simulink model "FieldOrientedController"  (R2020a)
settings: configuration reference "SLRT" (kept outside this file)
undefined symbols (not defined in the file): paramAdcAmperePerTransducerVolt, paramAdcTransducerVoltAtZeroAmpere, paramCurrentControlI, paramCurrentControlP, paramCurrentControlSatVoltage, paramEncoderCalibrationDuration, paramEncoderCalibrationMaxError, paramEncoderCalibrationVoltage, paramEncoderRotorPositionAtZeroCount, paramEncoderRotorPositionPerCount, paramOpenLoopVelocityAcceleration, paramOpenLoopVelocityToVoltsBias, paramOpenLoopVelocityToVoltsScalar, paramOverCurrentDuration, paramOverCurrentEnable, paramOverCurrentLimit, paramPwmCompareAtZeroVolt, paramPwmCompareMax, paramPwmComparePerVolt, paramVelocityControlI, paramVelocityControlP, paramVelocityControlSatCurrent, paramVelocityFilterCoeffDen, paramVelocityFilterCoeffNum, PolePairs, sampleTime
libraries: simulink x5
(part 2 of 2)

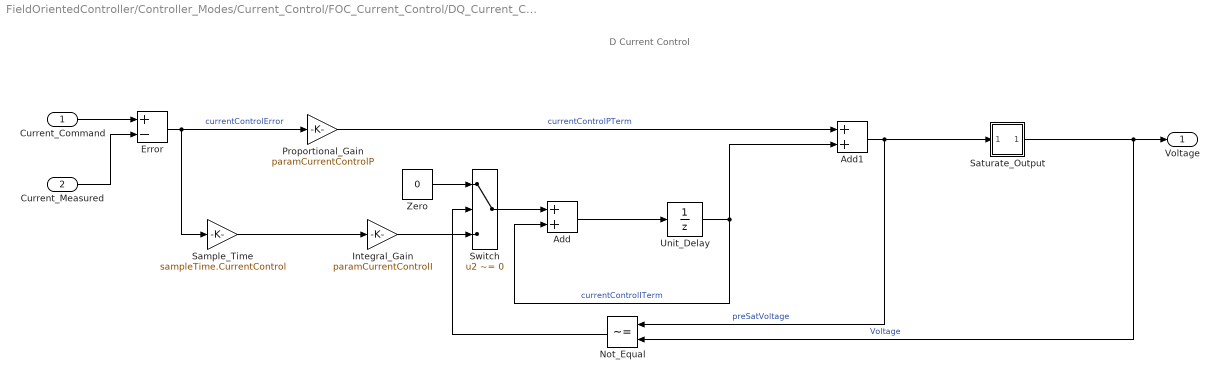
== system FieldOrientedController/Controller_Modes/Current_Control/FOC_Current_Control/DQ_Current_Control/D_Current_Control ==
  note: D Current Control
  Current_Command : Inport
  Current_Measured : Inport  Port=2
  Add : Sum
  Add1 : Sum
  Error : Sum  Inputs=+-
  Integral_Gain : Gain  Gain=paramCurrentControlI
      settings: AttributesFormatString=|
      | -----------------------------------
      | Gain = %<Gain>
  Not_Equal : RelationalOperator  Operator=~=  OutDataTypeStr=boolean  RndMeth=Nearest
  Proportional_Gain : Gain  Gain=paramCurrentControlP
      settings: AttributesFormatString=|
      | -----------------------------------
      | Gain = %<Gain>
  Sample_Time : Gain  Gain=sampleTime.CurrentControl
      settings: AttributesFormatString=|
      | -----------------------------------
      | Gain = %<Gain>
  Saturate_Output : Subsystem  mask(Saturate Magnitude){magnitudeLimit=paramCurrentControlSatVoltage}
      mask prompts: magnitudeLimit "Magnitude limit:"
      mask help:
      | Saturates input where:
      |    Upper limit =   Magnitude limit
      |    Lower limit = - Magnitude limit
      settings: AttributesFormatString=|
      | --------------------------------------------
      | Upper limit = %<magnitudeLimit>
      | Lower limit = -%<magnitudeLimit>
      mask Display: plot([0.15 0.85],[.5 .5],[.5 .5],[0.05 0.95],0.15+0.7*[0 .25 .75 1],0.05+0.9*[.25 .25 .75 .75]);
  Switch : Switch  Criteria=u2 ~= 0
  Unit_Delay : UnitDelay  SampleTime=-1  HasFrameUpgradeWarning=on
  Zero : Constant  Value=0  OutDataTypeStr=Inherit: Inherit via back propagation
  Voltage : Outport  VectorParamsAs1DForOutWhenUnconnected=off
  wires:
  Integral_Gain/1 -> Switch/3
  Unit_Delay/1 -> Add/2, Add1/2  "currentControlITerm"
  Sample_Time/1 -> Integral_Gain/1
  Add/1 -> Unit_Delay/1
  Not_Equal/1 -> Switch/2
  Proportional_Gain/1 -> Add1/1  "currentControlPTerm"
  Current_Measured/1 -> Error/2
  Switch/1 -> Add/1
  Saturate_Output/1(Out) -> Voltage/1, Not_Equal/2  "Voltage"
  Error/1 -> Proportional_Gain/1, Sample_Time/1  "currentControlError"
  Current_Command/1 -> Error/1
  Zero/1 -> Switch/1
  Add1/1 -> Not_Equal/1, Saturate_Output/1(In)  "preSatVoltage"

== system FieldOrientedController/Controller_Modes/Current_Control/FOC_Current_Control/DQ_Current_Control/Q_Current_Control ==
  note: Q Current Control
  Current_Command : Inport
  Current_Measured : Inport  Port=2
  Add : Sum
  Add1 : Sum
  Error : Sum  Inputs=+-
  Integral_Gain : Gain  Gain=paramCurrentControlI
      settings: AttributesFormatString=|
      | -----------------------------------
      | Gain = %<Gain>
  Not_Equal : RelationalOperator  Operator=~=  OutDataTypeStr=boolean  RndMeth=Nearest
  Proportional_Gain : Gain  Gain=paramCurrentControlP
      settings: AttributesFormatString=|
      | -----------------------------------
      | Gain = %<Gain>
  Sample_Time : Gain  Gain=sampleTime.CurrentControl
      settings: AttributesFormatString=|
      | -----------------------------------
      | Gain = %<Gain>
  Saturate_Output : Subsystem  mask(Saturate Magnitude){magnitudeLimit=paramCurrentControlSatVoltage}
      mask prompts: magnitudeLimit "Magnitude limit:"
      mask help:
      | Saturates input where:
      |    Upper limit =   Magnitude limit
      |    Lower limit = - Magnitude limit
      settings: AttributesFormatString=|
      | --------------------------------------------
      | Upper limit = %<magnitudeLimit>
      | Lower limit = -%<magnitudeLimit>
      mask Display: plot([0.15 0.85],[.5 .5],[.5 .5],[0.05 0.95],0.15+0.7*[0 .25 .75 1],0.05+0.9*[.25 .25 .75 .75]);
  Switch : Switch  Criteria=u2 ~= 0
  Unit_Delay : UnitDelay  SampleTime=-1  HasFrameUpgradeWarning=on
  Zero : Constant  Value=0  OutDataTypeStr=Inherit: Inherit via back propagation
  Voltage : Outport  VectorParamsAs1DForOutWhenUnconnected=off
  wires:
  Saturate_Output/1(Out) -> Voltage/1, Not_Equal/2  "Voltage"
  Add1/1 -> Not_Equal/1, Saturate_Output/1(In)  "preSatVoltage"
  Current_Measured/1 -> Error/2
  Unit_Delay/1 -> Add/2, Add1/2  "currentControlITerm"
  Proportional_Gain/1 -> Add1/1  "currentControlPTerm"
  Zero/1 -> Switch/1
  Error/1 -> Proportional_Gain/1, Sample_Time/1  "currentControlError"
  Sample_Time/1 -> Integral_Gain/1
  Current_Command/1 -> Error/1
  Add/1 -> Unit_Delay/1
  Integral_Gain/1 -> Switch/3
  Not_Equal/1 -> Switch/2
  Switch/1 -> Add/1

== system FieldOrientedController/Controller_Modes/Open_Loop_Velocity_Control/Open_Loop_Velocity_Control/Electrical_Velocity_To_Position/Mod_Two_Pi_Once ==
  note: Mod Two Pi Once
  X : Inport
  Add1 : Sum  Inputs=+-
  Add2 : Sum
  Greater_Than : RelationalOperator  OutDataTypeStr=boolean  RndMeth=Nearest
  Input_Range : SignalSpecification  OutMin=-4*pi  OutMax=4*pi
      settings: AttributesFormatString=|
      | -----------------------
      | Min = %<OutMin>
      | Max = %<OutMax>
  Less_Than : RelationalOperator  Operator=<  OutDataTypeStr=boolean  RndMeth=Nearest
  Output_Range : SignalSpecification  OutMin=0  OutMax=2*pi
      settings: AttributesFormatString=|
      | -----------------------
      | Min = %<OutMin>
      | Max = %<OutMax>
  Switch : Switch  Criteria=u2 ~= 0  InputSameDT=on
  Switch1 : Switch  Criteria=u2 ~= 0  InputSameDT=on
  Two_Pi : Constant  Value=2*pi  OutDataTypeStr=Inherit: Inherit via back propagation
  Two_Pi1 : Constant  Value=2*pi  OutDataTypeStr=Inherit: Inherit via back propagation
  Two_Pi2 : Constant  Value=2*pi  OutDataTypeStr=Inherit: Inherit via back propagation
  Zero : Constant  Value=0  OutDataTypeStr=Inherit: Inherit via back propagation
  Mod_X_Two_Pi : Outport  VectorParamsAs1DForOutWhenUnconnected=off
  wires:
  Output_Range/1 -> Mod_X_Two_Pi/1
  Zero/1 -> Less_Than/2
  Two_Pi2/1 -> Add2/2
  Add2/1 -> Switch1/1
  Less_Than/1 -> Switch1/2
  Switch1/1 -> Switch/3
  Two_Pi1/1 -> Greater_Than/2
  Two_Pi/1 -> Add1/2
  Add1/1 -> Switch/1
  Greater_Than/1 -> Switch/2
  X/1 -> Input_Range/1
  Switch/1 -> Output_Range/1
  Input_Range/1 -> Add1/1, Greater_Than/1, Add2/1, Less_Than/1, Switch1/3

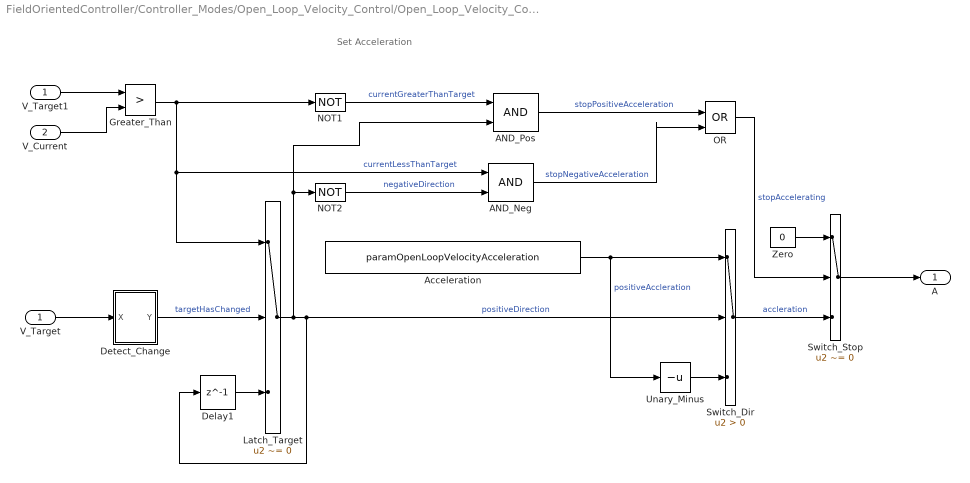
== system FieldOrientedController/Controller_Modes/Open_Loop_Velocity_Control/Open_Loop_Velocity_Control/Ramp_Velocity/Set_Acceleration ==
  note: Set Acceleration
  V_Target : Inport
  V_Current : Inport  Port=2
  AND_Neg : Logic  IconShape=distinctive  AllPortsSameDT=off  OutDataTypeStr=boolean
  AND_Pos : Logic  IconShape=distinctive  AllPortsSameDT=off  OutDataTypeStr=boolean
  Acceleration : Constant  Value=paramOpenLoopVelocityAcceleration  OutDataTypeStr=Inherit: Inherit via back propagation  SampleTime=-1
  Delay1 : Delay  DelayLength=1
  Detect_Change : Subsystem
  Greater_Than : RelationalOperator  Operator=>  OutDataTypeStr=boolean  RndMeth=Nearest
  Latch_Target : Switch  Criteria=u2 ~= 0
  NOT1 : Logic  Operator=NOT  IconShape=distinctive  AllPortsSameDT=off  OutDataTypeStr=boolean
  NOT2 : Logic  Operator=NOT  IconShape=distinctive  AllPortsSameDT=off  OutDataTypeStr=boolean
  OR : Logic  Operator=OR  IconShape=distinctive  AllPortsSameDT=off  OutDataTypeStr=boolean
  Switch_Dir : Switch  Criteria=u2 > Threshold
  Switch_Stop : Switch  Criteria=u2 ~= 0
  Unary_Minus : UnaryMinus
  V_Target1 : InportShadow
  Zero : Constant  Value=0  OutDataTypeStr=Inherit: Inherit via back propagation  SampleTime=-1
  A : Outport  VectorParamsAs1DForOutWhenUnconnected=off
  wires:
  AND_Neg/1 -> OR/2  "stopNegativeAcceleration"
  NOT2/1 -> AND_Neg/2  "negativeDirection"
  OR/1 -> Switch_Stop/2  "stopAccelerating"
  AND_Pos/1 -> OR/1  "stopPositiveAcceleration"
  NOT1/1 -> AND_Pos/1  "currentGreaterThanTarget"
  Zero/1 -> Switch_Stop/1
  Switch_Dir/1 -> Switch_Stop/3  "accleration"
  Switch_Stop/1 -> A/1
  Acceleration/1 -> Switch_Dir/1, Unary_Minus/1  "positiveAccleration"
  Unary_Minus/1 -> Switch_Dir/3
  Detect_Change/1(Y) -> Latch_Target/2  "targetHasChanged"
  V_Target/1 -> Detect_Change/1(X)
  V_Target1/1 -> Greater_Than/1
  V_Current/1 -> Greater_Than/2
  Delay1/1 -> Latch_Target/3
  Greater_Than/1 -> AND_Neg/1, Latch_Target/1, NOT1/1  "currentLessThanTarget"
  Latch_Target/1 -> Delay1/1, Switch_Dir/2, NOT2/1, AND_Pos/2  "positiveDirection"

== system FieldOrientedController/Controller_Modes/Current_Control/FOC_Current_Control/DQ_Current_Control/D_Current_Control/Saturate_Output ==
  note: Saturate Magnitude Library
  In : Inport
  Negate : UnaryMinus
  Saturation_Dynamic : simulink/Discontinuities/Saturation Dynamic  OutMin=[]  OutMax=[]  OutDataTypeStr=Inherit: Same as second input  OutDataType=fixdt(1, 16)  OutScaling=2^-10  DoSatur=off
  Saturation_Magntidue : Constant  Value=magnitudeLimit  OutDataTypeStr=Inherit: Inherit via back propagation
  Out : Outport  VectorParamsAs1DForOutWhenUnconnected=off
  wires:
  Saturation_Magntidue/1 -> Negate/1, Saturation_Dynamic/1
  Saturation_Dynamic/1 -> Out/1
  Negate/1 -> Saturation_Dynamic/3
  In/1 -> Saturation_Dynamic/2

== system FieldOrientedController/Controller_Modes/Current_Control/FOC_Current_Control/DQ_Current_Control/Q_Current_Control/Saturate_Output ==
  note: Saturate Magnitude Library
  In : Inport
  Negate : UnaryMinus
  Saturation_Dynamic : simulink/Discontinuities/Saturation Dynamic  OutMin=[]  OutMax=[]  OutDataTypeStr=Inherit: Same as second input  OutDataType=fixdt(1, 16)  OutScaling=2^-10  DoSatur=off
  Saturation_Magntidue : Constant  Value=magnitudeLimit  OutDataTypeStr=Inherit: Inherit via back propagation
  Out : Outport  VectorParamsAs1DForOutWhenUnconnected=off
  wires:
  Saturation_Magntidue/1 -> Negate/1, Saturation_Dynamic/1
  Saturation_Dynamic/1 -> Out/1
  Negate/1 -> Saturation_Dynamic/3
  In/1 -> Saturation_Dynamic/2

== system FieldOrientedController/Controller_Modes/Open_Loop_Velocity_Control/Open_Loop_Velocity_Control/Ramp_Velocity/Set_Acceleration/Detect_Change ==
  note: Detect Change
  X : Inport
  Add : Sum  Inputs=+-
  Delay : Delay  DelayLength=1
  Not_Equal_Zero : simulink/Logic and Bit Operations/Compare To Zero  relop=~=  OutDataTypeStr=boolean
  Y : Outport  VectorParamsAs1DForOutWhenUnconnected=off
  wires:
  Delay/1 -> Add/2
  Add/1 -> Not_Equal_Zero/1
  Not_Equal_Zero/1 -> Y/1
  X/1 -> Add/1, Delay/1

== stateflow chart FieldOrientedController/Controller_Modes/Over_Current_Detector/Detect_Over_Current_Error ==
  note: Detect Over Current Error
  note: If either Phase A Current (current[0]) or Phase B Current are above the threshold for a given duration, generate an error.
      | The error is reset when over current detection is disabled.
  state Error
    entry:
    error = true;
  state No_Error
    entry:
    error = false;
  state Wait_For_Reset
  (default) -> No_Error
  No_Error -> Error : [enableOverCurrentDetect && ...
      |  duration((phaseCurrentA >= paramOverCurrentLimit) || ...
      | (phaseCurrentB >= paramOverCurrentLimit))>paramOverCurrentDuration]
  Wait_For_Reset -> No_Error : [enableOverCurrentDetect]
  Error -> Wait_For_Reset : [~enableOverCurrentDetect]
  data: enableOverCurrentDetect input; phaseCurrentA input; phaseCurrentB input; error output boolean; paramOverCurrentDuration parameter; paramOverCurrentLimit parameter

== matlab function FieldOrientedController/EncoderToPositionAndVelocity/Position_Delta_To_Velocity/Rotor_Position_Delta_To_Velocity ==
  settings: fimath=|
      | fimath(...
      |     'RoundingMethod','Floor',...
      |     'OverflowAction','Wrap',...
      |     'ProductMode','KeepLSB',...
      |     'ProductWordLength',32,...
      |     'SumMode','KeepLSB',...
      |     'SumWordLength',32)
  data: positionDelta input; rotorVelocity output; positionDeltaBufferLength parameter; sampleFrequency parameter
function rotorVelocity = fcn(...                        %#codegen
                          positionDelta,...             % Input
                          positionDeltaBufferLength,... % Constant parameter
                          sampleFrequency)              % Constant parameter
% Copyright 2014 The MathWorks, Inc.

%% States
persistent positionDeltaBuffer;
persistent bufferIndex;

%% Constraints
assert(log2(positionDeltaBufferLength) == floor(log2(positionDeltaBufferLength)),...
    'Delay buffer must be a power of two.');

%% Initialize states
if isempty(positionDeltaBuffer)
    positionDeltaBuffer = ...
           zeros(positionDeltaBufferLength,1,...
                 'like', positionDelta);
    bufferIndex = int32(0);
end

%% Initialize constants
bufferIndexBitMask = positionDeltaBufferLength - 1;
reciprocalOfBufferLength = 1/positionDeltaBufferLength;

%% Step 
% Update delay buffer and index (MATLAB is one based indexing)
bufferIndex = bitand(bufferIndex+1, bufferIndexBitMask);
positionDeltaBuffer(bufferIndex+1) = positionDelta;

% Calculate velocity
positionDeltaSum = sum(positionDeltaBuffer);
rotorVelocity = positionDeltaSum * sampleFrequency * reciprocalOfBufferLength;
